simulink model "reverberation"  (R2020a)
settings: Solver=VariableStepAuto  StartTime=0.0  StopTime=50  RelTol=1e-3
libraries: dspvision x1, dspobslib x1
settings Model: Creator=XPS 15  LastModifiedBy=XPS 15

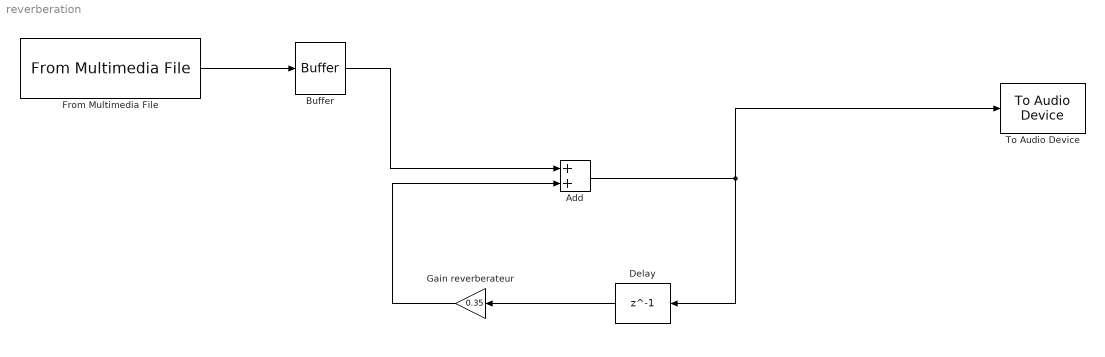
== system reverberation ==
  Add : Sum
  Buffer : Buffer  N=24000  OutputFrames=off
  Delay : Delay  DelayLength=1  DelayLengthUpperLimit=5000
  From Multimedia File : dspvision/From Multimedia File  inputFilename=C:\Users\XPS 15\Desktop\L05 Sorbonne\images\Son\Projet\les-abranis-mel-iyi-paroles-R6wh6KdZLxw.mp3  readRange=[1 Inf]  loop=on  numPlays=inf  outputStreams=Audio only  videoDataType=single  audioDataType=double  inheritSampleTime=on  userDefinedSampleTime=1/30  noAudioOutput=off  isIntensityVideo=off  fourcc=RGB  colorVideoFormat=Separate color signals  outputEOF=off  dataOrg=Column-major  audioFrameSize=1  computeAudioFrameSize=off  outSamplingMode=Sample based
  Gain reverberateur : Gain  Gain=0.35
  To Audio Device : dspobslib/To Audio Device  deviceName=Default  inheritSampleRate=on  sampleRate=44100  deviceDatatype=Determine from input data type  autoBufferSize=on  bufferSize=4096  queueDuration=1.0  defaultOutputChannelMapping=on  outputChannelMapping=1:2  outputNumUnderrunSamples=off
      settings: SourceProductBaseCode=DS
  wires:
  Delay/1 -> Gain reverberateur/1
  Add/1 -> Delay/1, To Audio Device/1
  Gain reverberateur/1 -> Add/2
  Buffer/1 -> Add/1
  From Multimedia File/1 -> Buffer/1
